simulink model "ddc_bpm_476_066"  (Simulink 7.8)
settings: Solver=ode45  StartTime=0.0  StopTime=2e-3  RelTol=1e-3
undefined symbols (not defined in the file): decim_factor_poly_35, dt_sim, frev_476, Fs_adc, n_ch, n_ovs, R_fofb, R_sec, R_sec_cfir, R_sec_pfir, R_tbt, xlipgetpartsetting
libraries: xbsIndex_r4 x1408, simulink x7
(part 5 of 11)

== system ddc_bpm_476_066/K_monit_mult3/Cast_truncate1 ==
  In1 : Inport
  Reinterpret : xbsIndex_r4/Reinterpret  force_arith_type=on  arith_type="Signed  (2's comp)"  force_bin_pt=on  bin_pt=0  block_type=reinterpret
  Slice : xbsIndex_r4/Slice  nbits=26  boolean_output=off  mode=Upper Bit Location + Width  bit1=0  base1=MSB of Input  bit0=0  base0=LSB of Input  dbl_ovrd=off  block_type=slice
  Out1 : Outport
  wires:
  Slice/1 -> Reinterpret/1
  Reinterpret/1 -> Out1/1
  In1/1 -> Slice/1

== system ddc_bpm_476_066/K_monit_mult4/Cast_truncate1 ==
  In1 : Inport
  Reinterpret : xbsIndex_r4/Reinterpret  force_arith_type=on  arith_type="Signed  (2's comp)"  force_bin_pt=on  bin_pt=0  block_type=reinterpret
  Slice : xbsIndex_r4/Slice  nbits=26  boolean_output=off  mode=Upper Bit Location + Width  bit1=0  base1=MSB of Input  bit0=0  base0=LSB of Input  dbl_ovrd=off  block_type=slice
  Out1 : Outport
  wires:
  Slice/1 -> Reinterpret/1
  Reinterpret/1 -> Out1/1
  In1/1 -> Slice/1

== system ddc_bpm_476_066/K_monit_mult5/Cast_truncate1 ==
  In1 : Inport
  Reinterpret : xbsIndex_r4/Reinterpret  force_arith_type=on  arith_type="Signed  (2's comp)"  force_bin_pt=on  bin_pt=0  block_type=reinterpret
  Slice : xbsIndex_r4/Slice  nbits=26  boolean_output=off  mode=Upper Bit Location + Width  bit1=0  base1=MSB of Input  bit0=0  base0=LSB of Input  dbl_ovrd=off  block_type=slice
  Out1 : Outport
  wires:
  Slice/1 -> Reinterpret/1
  Reinterpret/1 -> Out1/1
  In1/1 -> Slice/1

== system ddc_bpm_476_066/K_tbt_mult/Cast_truncate1 ==
  In1 : Inport
  Reinterpret : xbsIndex_r4/Reinterpret  force_arith_type=on  arith_type="Signed  (2's comp)"  force_bin_pt=on  bin_pt=0  block_type=reinterpret
  Slice : xbsIndex_r4/Slice  nbits=26  boolean_output=off  mode=Upper Bit Location + Width  bit1=0  base1=MSB of Input  bit0=0  base0=LSB of Input  dbl_ovrd=off  block_type=slice
  Out1 : Outport
  wires:
  Slice/1 -> Reinterpret/1
  Reinterpret/1 -> Out1/1
  In1/1 -> Slice/1

== system ddc_bpm_476_066/K_tbt_mult1/Cast_truncate1 ==
  In1 : Inport
  Reinterpret : xbsIndex_r4/Reinterpret  force_arith_type=on  arith_type="Signed  (2's comp)"  force_bin_pt=on  bin_pt=0  block_type=reinterpret
  Slice : xbsIndex_r4/Slice  nbits=26  boolean_output=off  mode=Upper Bit Location + Width  bit1=0  base1=MSB of Input  bit0=0  base0=LSB of Input  dbl_ovrd=off  block_type=slice
  Out1 : Outport
  wires:
  Slice/1 -> Reinterpret/1
  Reinterpret/1 -> Out1/1
  In1/1 -> Slice/1

== system ddc_bpm_476_066/K_tbt_mult2/Cast_truncate1 ==
  In1 : Inport
  Reinterpret : xbsIndex_r4/Reinterpret  force_arith_type=on  arith_type="Signed  (2's comp)"  force_bin_pt=on  bin_pt=0  block_type=reinterpret
  Slice : xbsIndex_r4/Slice  nbits=26  boolean_output=off  mode=Upper Bit Location + Width  bit1=0  base1=MSB of Input  bit0=0  base0=LSB of Input  dbl_ovrd=off  block_type=slice
  Out1 : Outport
  wires:
  Slice/1 -> Reinterpret/1
  Reinterpret/1 -> Out1/1
  In1/1 -> Slice/1

== system ddc_bpm_476_066/Ksum_fofb_mult4/Cast_truncate1 ==
  In1 : Inport
  Reinterpret : xbsIndex_r4/Reinterpret  force_arith_type=on  arith_type="Signed  (2's comp)"  force_bin_pt=on  bin_pt=20  block_type=reinterpret
  Slice : xbsIndex_r4/Slice  nbits=26  boolean_output=off  mode=Upper Bit Location + Width  bit1=0  base1=MSB of Input  bit0=0  base0=LSB of Input  dbl_ovrd=off  block_type=slice
  Out1 : Outport
  wires:
  Slice/1 -> Reinterpret/1
  Reinterpret/1 -> Out1/1
  In1/1 -> Slice/1

== system ddc_bpm_476_066/Ksum_monit_1_mult1/Cast_truncate1 ==
  In1 : Inport
  Reinterpret : xbsIndex_r4/Reinterpret  force_arith_type=on  arith_type="Signed  (2's comp)"  force_bin_pt=on  bin_pt=20  block_type=reinterpret
  Slice : xbsIndex_r4/Slice  nbits=26  boolean_output=off  mode=Upper Bit Location + Width  bit1=0  base1=MSB of Input  bit0=0  base0=LSB of Input  dbl_ovrd=off  block_type=slice
  Out1 : Outport
  wires:
  Slice/1 -> Reinterpret/1
  Reinterpret/1 -> Out1/1
  In1/1 -> Slice/1

== system ddc_bpm_476_066/Ksum_monit_mult2/Cast_truncate1 ==
  In1 : Inport
  Reinterpret : xbsIndex_r4/Reinterpret  force_arith_type=on  arith_type="Signed  (2's comp)"  force_bin_pt=on  bin_pt=20  block_type=reinterpret
  Slice : xbsIndex_r4/Slice  nbits=26  boolean_output=off  mode=Upper Bit Location + Width  bit1=0  base1=MSB of Input  bit0=0  base0=LSB of Input  dbl_ovrd=off  block_type=slice
  Out1 : Outport
  wires:
  Slice/1 -> Reinterpret/1
  Reinterpret/1 -> Out1/1
  In1/1 -> Slice/1

== system ddc_bpm_476_066/Ksum_tbt_mult3/Cast_truncate1 ==
  In1 : Inport
  Reinterpret : xbsIndex_r4/Reinterpret  force_arith_type=on  arith_type="Signed  (2's comp)"  force_bin_pt=on  bin_pt=20  block_type=reinterpret
  Slice : xbsIndex_r4/Slice  nbits=26  boolean_output=off  mode=Upper Bit Location + Width  bit1=0  base1=MSB of Input  bit0=0  base0=LSB of Input  dbl_ovrd=off  block_type=slice
  Out1 : Outport
  wires:
  Slice/1 -> Reinterpret/1
  Reinterpret/1 -> Out1/1
  In1/1 -> Slice/1

== system ddc_bpm_476_066/Mixer/CMixer_0 ==
  din_q : Inport
  din_i : Inport  Port=2
  en : Inport  Port=3
  dds_valid : Inport  Port=4
  dds_msine : Inport  Port=5
  dds_cosine : Inport  Port=6
  ch_in : Inport  Port=7
  ComplexMult : xbsIndex_r4/Complex Multiplier 5.0   hasatlast=off  hasatuser=off  atuserwidth=1  hasbtlast=off  hasbtuser=on  btuserwidth=ceil(log2(n_ovs))  multtype=Use_Mults  optimizegoal=Performance  flowcontrol=NonBlocking  outputwidth=24  roundmode=Truncate  hasctrltlast=off  hasctrltuser=off  ctrltuserwidth=1  outtlastbehv=Null  latencyconfig=Automatic  minimumlatency=34  aclken=off  aresetn=off  trim_axipin_name=on  aportwidth=63  bportwidth=63  ip_name=Complex Multiplier  ip_version=5.0  dsptool_ready=true  ipcore_usecache=true  ipcore_useipmodelcache=true  ipcore_verbose=false  ipcore_latency_parameter='minimumlatency'  wrapper_available=true  port_translation_map={ 'aclken' => 'en', 'aresetn' => 'rst'}  structural_sim=false  block_type=cmpy_v5_0
  Convert1 : xbsIndex_r4/Convert  gui_display_data_type=Fixed-point  arith_type="Signed  (2's comp)"  n_bits=24  bin_pt=22  float_type=Single  exp_bits=8  fraction_bits=24  quantization=Truncate  overflow=Flag as error  en=off  latency=0  dbl_ovrd=off  pipeline=off  block_type=convert
  Convert2 : xbsIndex_r4/Convert  gui_display_data_type=Fixed-point  arith_type="Signed  (2's comp)"  n_bits=24  bin_pt=22  float_type=Single  exp_bits=8  fraction_bits=24  quantization=Truncate  overflow=Flag as error  en=off  latency=0  dbl_ovrd=off  pipeline=off  block_type=convert
  DataReg_En : Subsystem
  DataReg_En1 : Subsystem
  Delay : xbsIndex_r4/Delay  rst=off  infoeditControl=Selection of Reset will increase slice count due to use of real FFs and instead of SRLs  en=off  latency=0  dbl_ovrd=off  reg_retiming=off  block_type=delay
      settings: infoedit=Hardware notes: A delay line is a chain, each link of which is an SRL16 followed by a flip-flop. If register retiming is enabled, the delay line is a chain of flip-flops.  xl_area=[7 14 0 0 0 0 0]  block_version=VER_STRING_GOES_HERE
  Delay1 : xbsIndex_r4/Delay  rst=off  infoeditControl=Selection of Reset will increase slice count due to use of real FFs and instead of SRLs  en=off  latency=0  dbl_ovrd=off  reg_retiming=off  block_type=delay
      settings: infoedit=Hardware notes: A delay line is a chain, each link of which is an SRL16 followed by a flip-flop. If register retiming is enabled, the delay line is a chain of flip-flops.  xl_area=[7 14 0 0 0 0 0]  block_version=VER_STRING_GOES_HERE
  Register{,1..5} (6 alike) : xbsIndex_r4/Register  init=0  rst=off  en=on  dbl_ovrd=off  block_type=register
      settings: block_version=VER_STRING_GOES_HERE
  Register6 : xbsIndex_r4/Register  init=0  rst=off  en=off  dbl_ovrd=off  block_type=register
      settings: block_version=VER_STRING_GOES_HERE
  Reinterpret : xbsIndex_r4/Reinterpret  force_arith_type=off  arith_type=Unsigned  force_bin_pt=off  bin_pt=22  block_type=reinterpret
  Reinterpret1 : xbsIndex_r4/Reinterpret  force_arith_type=off  arith_type=Unsigned  force_bin_pt=off  bin_pt=22  block_type=reinterpret
  Terminator : Terminator
  Q_out : Outport
  I_out : Outport  Port=2
  ch_out : Outport  Port=3
  vout : Outport  Port=4
  wires:
  DataReg_En/1(Dout) -> Delay/1
  DataReg_En1/1(Dout) -> Delay1/1
  dds_cosine/1 -> Register1/1
  dds_msine/1 -> Register2/1
  Register1/1 -> ComplexMult/3  "a_r"
  Register5/1 -> Q_out/1
  Register2/1 -> ComplexMult/2  "a_i"
  ComplexMult/2 -> Reinterpret/1
  ComplexMult/3 -> Reinterpret1/1
  ComplexMult/1 -> Register3/2, Register4/2, Register5/2, Register6/1
  Delay1/1 -> ComplexMult/6  "b_r"
  Delay/1 -> ComplexMult/5  "b_i"
  DataReg_En/2(Valid) -> ComplexMult/4
  Register4/1 -> I_out/1
  Convert1/1 -> Register4/1
  Convert2/1 -> Register5/1
  Reinterpret/1 -> Convert2/1
  Reinterpret1/1 -> Convert1/1
  dds_valid/1 -> Register1/2, Register2/2, ComplexMult/1
  din_q/1 -> DataReg_En/1(Din)
  din_i/1 -> DataReg_En1/1(Din)
  en/1 -> DataReg_En/2(en), DataReg_En1/2(en), Register/2
  ch_in/1 -> Register/1
  Register/1 -> ComplexMult/7
  Register3/1 -> ch_out/1
  ComplexMult/4 -> Register3/1
  Register6/1 -> vout/1
  DataReg_En1/2(Valid) -> Terminator/1

== system ddc_bpm_476_066/Mixer/CMixer_1 ==
  din_q : Inport
  din_i : Inport  Port=2
  en : Inport  Port=3
  dds_valid : Inport  Port=4
  dds_msine : Inport  Port=5
  dds_cosine : Inport  Port=6
  ch_in : Inport  Port=7
  ComplexMult : xbsIndex_r4/Complex Multiplier 5.0   hasatlast=off  hasatuser=off  atuserwidth=1  hasbtlast=off  hasbtuser=on  btuserwidth=ceil(log2(n_ovs))  multtype=Use_Mults  optimizegoal=Performance  flowcontrol=NonBlocking  outputwidth=24  roundmode=Truncate  hasctrltlast=off  hasctrltuser=off  ctrltuserwidth=1  outtlastbehv=Null  latencyconfig=Automatic  minimumlatency=34  aclken=off  aresetn=off  trim_axipin_name=on  aportwidth=63  bportwidth=63  ip_name=Complex Multiplier  ip_version=5.0  dsptool_ready=true  ipcore_usecache=true  ipcore_useipmodelcache=true  ipcore_verbose=false  ipcore_latency_parameter='minimumlatency'  wrapper_available=true  port_translation_map={ 'aclken' => 'en', 'aresetn' => 'rst'}  structural_sim=false  block_type=cmpy_v5_0
  Convert1 : xbsIndex_r4/Convert  gui_display_data_type=Fixed-point  arith_type="Signed  (2's comp)"  n_bits=24  bin_pt=22  float_type=Single  exp_bits=8  fraction_bits=24  quantization=Truncate  overflow=Flag as error  en=off  latency=0  dbl_ovrd=off  pipeline=off  block_type=convert
  Convert2 : xbsIndex_r4/Convert  gui_display_data_type=Fixed-point  arith_type="Signed  (2's comp)"  n_bits=24  bin_pt=22  float_type=Single  exp_bits=8  fraction_bits=24  quantization=Truncate  overflow=Flag as error  en=off  latency=0  dbl_ovrd=off  pipeline=off  block_type=convert
  DataReg_En : Subsystem
  DataReg_En1 : Subsystem
  Delay : xbsIndex_r4/Delay  rst=off  infoeditControl=Selection of Reset will increase slice count due to use of real FFs and instead of SRLs  en=off  latency=0  dbl_ovrd=off  reg_retiming=off  block_type=delay
      settings: infoedit=Hardware notes: A delay line is a chain, each link of which is an SRL16 followed by a flip-flop. If register retiming is enabled, the delay line is a chain of flip-flops.  xl_area=[7 14 0 0 0 0 0]  block_version=VER_STRING_GOES_HERE
  Delay1 : xbsIndex_r4/Delay  rst=off  infoeditControl=Selection of Reset will increase slice count due to use of real FFs and instead of SRLs  en=off  latency=0  dbl_ovrd=off  reg_retiming=off  block_type=delay
      settings: infoedit=Hardware notes: A delay line is a chain, each link of which is an SRL16 followed by a flip-flop. If register retiming is enabled, the delay line is a chain of flip-flops.  xl_area=[7 14 0 0 0 0 0]  block_version=VER_STRING_GOES_HERE
  Register{,1..5} (6 alike) : xbsIndex_r4/Register  init=0  rst=off  en=on  dbl_ovrd=off  block_type=register
      settings: block_version=VER_STRING_GOES_HERE
  Register6 : xbsIndex_r4/Register  init=0  rst=off  en=off  dbl_ovrd=off  block_type=register
      settings: block_version=VER_STRING_GOES_HERE
  Reinterpret : xbsIndex_r4/Reinterpret  force_arith_type=off  arith_type=Unsigned  force_bin_pt=off  bin_pt=22  block_type=reinterpret
  Reinterpret1 : xbsIndex_r4/Reinterpret  force_arith_type=off  arith_type=Unsigned  force_bin_pt=off  bin_pt=22  block_type=reinterpret
  Terminator : Terminator
  Q_out : Outport
  I_out : Outport  Port=2
  ch_out : Outport  Port=3
  vout : Outport  Port=4
  wires:
  DataReg_En/1(Dout) -> Delay/1
  DataReg_En1/1(Dout) -> Delay1/1
  dds_cosine/1 -> Register1/1
  dds_msine/1 -> Register2/1
  Register1/1 -> ComplexMult/3  "a_r"
  Register5/1 -> Q_out/1
  Register2/1 -> ComplexMult/2  "a_i"
  ComplexMult/2 -> Reinterpret/1
  ComplexMult/3 -> Reinterpret1/1
  ComplexMult/1 -> Register3/2, Register4/2, Register5/2, Register6/1
  Delay1/1 -> ComplexMult/6  "b_r"
  Delay/1 -> ComplexMult/5  "b_i"
  DataReg_En/2(Valid) -> ComplexMult/4
  Register4/1 -> I_out/1
  Convert1/1 -> Register4/1
  Convert2/1 -> Register5/1
  Reinterpret/1 -> Convert2/1
  Reinterpret1/1 -> Convert1/1
  dds_valid/1 -> Register1/2, Register2/2, ComplexMult/1
  din_q/1 -> DataReg_En/1(Din)
  din_i/1 -> DataReg_En1/1(Din)
  en/1 -> DataReg_En/2(en), DataReg_En1/2(en), Register/2
  ch_in/1 -> Register/1
  Register/1 -> ComplexMult/7
  Register3/1 -> ch_out/1
  ComplexMult/4 -> Register3/1
  Register6/1 -> vout/1
  DataReg_En1/2(Valid) -> Terminator/1

== system ddc_bpm_476_066/Mixer/ST5 ==
  In : Inport
  Display : Display
  Sample Time : xbsIndex_r4/Sample Time  block_type=sampletime
      settings: infoedit="The Sample Time block reports the normalized sample period of its input.  A signal's normalized sample period is not equivalent to its Simulink absolute sample period.<br><br>Hardware notes: This block is implemented as a constant in hardware."
  out : xbsIndex_r4/Gateway Out  inherit_from_input=on  hdl_port=off  timing_constraint=Data Rate  locs_specified=off  LOCs={}  UseAsDAC=off  DACChannel='1'  block_type=gatewayout
      settings: infoedit="Gateway out block.  Converts Xilinx fixed-point or floating-point type inputs into ouputs of type Simulink integer, single, double, or fixed point.<br><br>Hardware notes:  In hardware these blocks become top level output ports or are discarded, depending on how they are configured."
  wires:
  out/1 -> Display/1
  Sample Time/1 -> out/1
  In/1 -> Sample Time/1

== system ddc_bpm_476_066/Mixer/TDDM_Mixer ==
  mix0_q_in : Inport
  mix0_i_in : Inport  Port=2
  mix0_ch_in : Inport  Port=3
  mix1_q_in : Inport  Port=4
  mix1_i_in : Inport  Port=5
  mix1_ch_in : Inport  Port=6
  TDDM_Mixer0_i : Subsystem
  TDDM_Mixer0_q : Subsystem
  TDDM_Mixer1_i : Subsystem
  TDDM_Mixer1_q : Subsystem
  Terminator{,1..3} (4 alike) : Terminator
  mix_ch0_q_out : Outport
  mix_ch1_q_out : Outport  Port=2
  mix_ch2_q_out : Outport  Port=3
  mix_ch3_q_out : Outport  Port=4
  mix_ch0_i_out : Outport  Port=5
  mix_ch1_i_out : Outport  Port=6
  mix_ch2_i_out : Outport  Port=7
  mix_ch3_i_out : Outport  Port=8
  wires:
  mix0_q_in/1 -> TDDM_Mixer0_q/1(din)
  mix0_ch_in/1 -> TDDM_Mixer0_q/2(ch_in), TDDM_Mixer0_i/2(ch_in)
  mix0_i_in/1 -> TDDM_Mixer0_i/1(din)
  mix1_q_in/1 -> TDDM_Mixer1_q/1(din)
  mix1_ch_in/1 -> TDDM_Mixer1_q/2(ch_in), TDDM_Mixer1_i/2(ch_in)
  mix1_i_in/1 -> TDDM_Mixer1_i/1(din)
  TDDM_Mixer0_q/1(dout_ch0) -> mix_ch0_q_out/1
  TDDM_Mixer0_q/2(dout_ch1) -> mix_ch1_q_out/1
  TDDM_Mixer0_i/1(dout_ch0) -> mix_ch0_i_out/1
  TDDM_Mixer0_i/2(dout_ch1) -> mix_ch1_i_out/1
  TDDM_Mixer1_q/1(dout_ch0) -> mix_ch2_q_out/1
  TDDM_Mixer1_q/2(dout_ch1) -> mix_ch3_q_out/1
  TDDM_Mixer1_i/1(dout_ch0) -> mix_ch2_i_out/1
  TDDM_Mixer1_i/2(dout_ch1) -> mix_ch3_i_out/1
  TDDM_Mixer0_i/3(ch_out) -> Terminator/1
  TDDM_Mixer0_q/3(ch_out) -> Terminator1/1
  TDDM_Mixer1_i/3(ch_out) -> Terminator2/1
  TDDM_Mixer1_q/3(ch_out) -> Terminator3/1

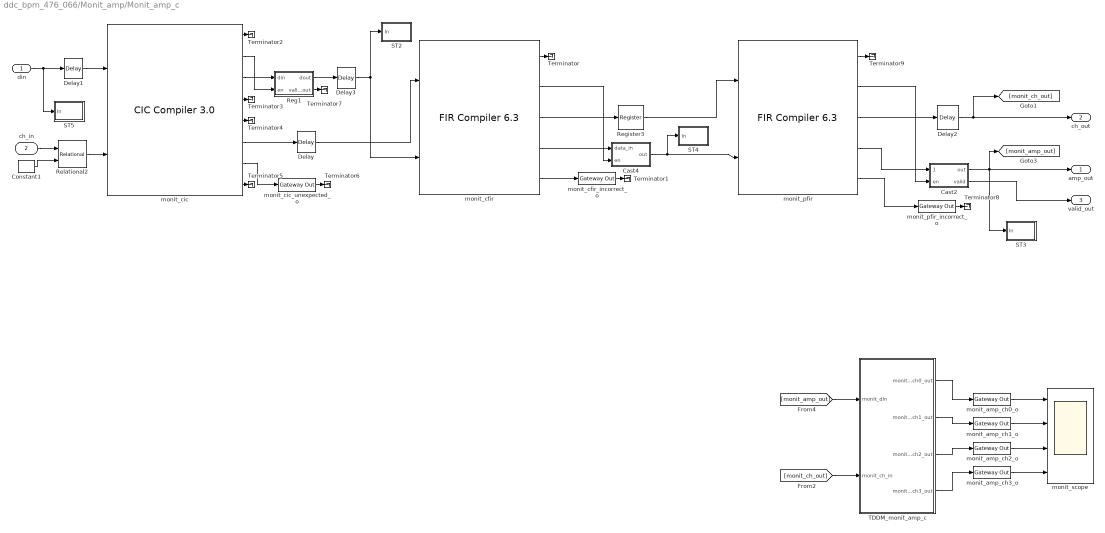
== system ddc_bpm_476_066/Monit_amp/Monit_amp_c ==
  din : Inport
  ch_in : Inport  Port=2
  Cast2 : Subsystem
  Cast4 : Subsystem
  Constant1 : xbsIndex_r4/Constant  const=2  gui_display_data_type=Fixed-point  arith_type=Unsigned  n_bits=2  bin_pt=0  preci_type=Single  exp_width=8  frac_width=24  explicit_period=off  period=1  equ=P=C  opselect=C  inp2=PCIN>>17  opr=+  inp1=P  carry=CIN  dbl_ovrd=off  block_type=constant
  Delay : xbsIndex_r4/Delay  rst=off  infoeditControl=Selection of Reset will increase slice count due to use of real FFs and instead of SRLs  en=off  latency=3  dbl_ovrd=off  reg_retiming=off  block_type=delay
  Delay1 : xbsIndex_r4/Delay  rst=off  infoeditControl=Selection of Reset will increase slice count due to use of real FFs and instead of SRLs  en=off  latency=3  dbl_ovrd=off  reg_retiming=off  block_type=delay
  Delay2 : xbsIndex_r4/Delay  rst=off  infoeditControl=Selection of Reset will increase slice count due to use of real FFs and instead of SRLs  en=off  latency=1  dbl_ovrd=off  reg_retiming=off  block_type=delay
  Delay3 : xbsIndex_r4/Delay  rst=off  infoeditControl=Selection of Reset will increase slice count due to use of real FFs and instead of SRLs  en=off  latency=2  dbl_ovrd=off  reg_retiming=off  block_type=delay
  Reg1 : Subsystem
  Register3 : xbsIndex_r4/Register  init=0  rst=off  en=off  dbl_ovrd=off  block_type=register
      settings: xl_area=[0, 0, 0, 0, 0, 0, 0]  block_version=VER_STRING_GOES_HERE
  Relational2 : xbsIndex_r4/Relational  mode=a=b  en=off  latency=4  dbl_ovrd=off  block_type=relational
  ST2 : Subsystem
  ST3 : Subsystem
  ST4 : Subsystem
  ST5 : Subsystem
  TDDM_monit_amp_c : Subsystem
  Terminator{,1..9} (10 alike) : Terminator
  monit_amp_ch0_o : xbsIndex_r4/Gateway Out  inherit_from_input=on  hdl_port=on  timing_constraint=Data Rate  locs_specified=off  LOCs={}  UseAsDAC=off  DACChannel='1'  block_type=gatewayout
      settings: infoedit="Gateway out block.  Converts Xilinx fixed-point or floating-point type inputs into ouputs of type Simulink integer, single, double, or fixed point.<br><br>Hardware notes:  In hardware these blocks become top level output ports or are discarded, depending on how they are configured."
  monit_amp_ch1_o : xbsIndex_r4/Gateway Out  inherit_from_input=on  hdl_port=on  timing_constraint=Data Rate  locs_specified=off  LOCs={}  UseAsDAC=off  DACChannel='1'  block_type=gatewayout
      settings: infoedit="Gateway out block.  Converts Xilinx fixed-point or floating-point type inputs into ouputs of type Simulink integer, single, double, or fixed point.<br><br>Hardware notes:  In hardware these blocks become top level output ports or are discarded, depending on how they are configured."
  monit_amp_ch2_o : xbsIndex_r4/Gateway Out  inherit_from_input=on  hdl_port=on  timing_constraint=Data Rate  locs_specified=off  LOCs={}  UseAsDAC=off  DACChannel='1'  block_type=gatewayout
      settings: infoedit="Gateway out block.  Converts Xilinx fixed-point or floating-point type inputs into ouputs of type Simulink integer, single, double, or fixed point.<br><br>Hardware notes:  In hardware these blocks become top level output ports or are discarded, depending on how they are configured."
  monit_amp_ch3_o : xbsIndex_r4/Gateway Out  inherit_from_input=on  hdl_port=on  timing_constraint=Data Rate  locs_specified=off  LOCs={}  UseAsDAC=off  DACChannel='1'  block_type=gatewayout
      settings: infoedit="Gateway out block.  Converts Xilinx fixed-point or floating-point type inputs into ouputs of type Simulink integer, single, double, or fixed point.<br><br>Hardware notes:  In hardware these blocks become top level output ports or are discarded, depending on how they are configured."
  monit_cfir : xbsIndex_r4/FIR Compiler 6.3   coefficientvector=hcfir_sec.Numerator  coefficient_sets=1  coefficient_reload=off  filter_type=Decimation  rate_change_type=Integer  interpolation_rate=1  decimation_rate=R_sec_cfir  zero_pack_factor=1  channel_sequence=Basic  number_channels=4  pattern_list='P4-0,P4-1,P4-2,P4-3,P4-4'  number_paths=1  ratespecification=Hardware_Oversampling_Rate  sampleperiod=1  hardwareoversamplingrate=R_fofb*R_sec*n_ovs/n_ch  coefficient_sign=Signed  quantization=Quantize_Only  coefficient_width=16  bestprecision=on  coefficient_fractional_bits=15  coefficient_structure=Inferred  output_rounding_mode=Convergent_Rounding_to_Even  output_width=25  filter_architecture=Systolic_Multiply_Accumulate  optimization_goal=Area  data_buffer_type=Automatic  coefficient_buffer_type=Automatic  input_buffer_type=Automatic  output_buffer_type=Automatic  preference_for_other_storage=Automatic  multi_column_support=Automatic  columnconfig='1'  inter_column_pipe_length=4  data_has_tlast=Not_Required  m_data_has_tready=off  s_data_has_fifo=off  s_data_has_tuser=Chan_ID_Field  m_data_has_tuser=Chan_ID_Field  s_config_sync_mode=On_Vector  s_config_method=Single  num_reload_slots=1  has_aclken=off  has_aresetn=off  infoeditControl=ARESETn must be asserted for a minmum of 2 cycles  trim_axipin_name=on  passband_min=0.0  passband_max=0.5  stopband_min=0.5  stopband_max=1.0  filter_selection=1  gui_behaviour=Sysgen_GUI  data_sign=Signed  data_width=16  data_fractional_bits=0  data_tuser_width=1  wrapper_available=true  ip_wrap_arbitrary_binary_point=true  simulation_type=external_xfix  simulation_model=firv6_3_CModel:firv6_3_cmodel  ip_name=FIR Compiler  ip_version=6.3  dsptool_ready=true  ipcore_usecache=true  ipcore_useipmodelcache=true  ipcore_xco_need_fpga_part=true  port_translation_map={ 'aclken' => 'en', 'aresetn' => 'rst' }  run_core_at_system_period=true  ipcore_fpga_part=xlipgetpartsetting(gcb, {'virtex6', 'xc6vlx75t', '-3', 'ff784'})  block_type=fir_compiler_v6_3
      settings: infoedit=Maximum Possible : Maximizes oversampling rate. Abstracted input handshake (no s_data_tvalid) and automatic rate propagation.<br>Hardware Oversampling Rate : Specifies oversampling rate relative to the input sample period. Abstracted input handshake (no s_data_tvalid) and automatic rate propagation.<br>Sample Period : Specifies absolute oversampling rate. No input handshake abstraction (exposes s_data_tvalid) and no rate propagation.
  monit_cfir_incorrect_o : xbsIndex_r4/Gateway Out  inherit_from_input=on  hdl_port=on  timing_constraint=Data Rate  locs_specified=off  LOCs={}  UseAsDAC=off  DACChannel='1'  block_type=gatewayout
      settings: infoedit="Gateway out block.  Converts Xilinx fixed-point or floating-point type inputs into ouputs of type Simulink integer, single, double, or fixed point.<br><br>Hardware notes:  In hardware these blocks become top level output ports or are discarded, depending on how they are configured."
  monit_cic : xbsIndex_r4/CIC Compiler 3.0   filter_type=Decimation  number_of_stages=3  differential_delay=2  number_of_channels=4  sample_rate_changes=Fixed  fixed_or_initial_rate=R_sec  minimum_rate=2500  maximum_rate=2500  ratespecification=Hardware_Oversampling_Rate  sampleperiod=1  hardwareoversamplingrate=R_fofb*n_ovs/n_ch  quantization=Full_Precision  output_data_width=55  use_xtreme_dsp_slice=on  use_streaming_interface=on  has_aclken=off  has_aresetn=off  has_dout_tready=off  trim_axipin_name=on  gui_behaviour=Sysgen_GUI  input_data_width=18  ip_name=CIC Compiler  ip_version=3.0  dsptool_ready=true  wrapper_available=true  port_translation_map={ 'aclken' => 'en', 'aresetn' => 'rst' }  ipcore_xco_need_fpga_part=true  ipcore_fpga_part=xlipgetpartsetting(gcb, {'virtex7', 'xc7v1500t', '-2', 'fhg1157'})  ipcore_verbose=false  block_type=cic_compiler_v3_0
  monit_cic_unexpected_o : xbsIndex_r4/Gateway Out  inherit_from_input=on  hdl_port=on  timing_constraint=Data Rate  locs_specified=off  LOCs={}  UseAsDAC=off  DACChannel='1'  block_type=gatewayout
      settings: infoedit="Gateway out block.  Converts Xilinx fixed-point or floating-point type inputs into ouputs of type Simulink integer, single, double, or fixed point.<br><br>Hardware notes:  In hardware these blocks become top level output ports or are discarded, depending on how they are configured."
  monit_pfir : xbsIndex_r4/FIR Compiler 6.3   coefficientvector=hpfir_sec.Numerator  coefficient_sets=1  coefficient_reload=off  filter_type=Decimation  rate_change_type=Integer  interpolation_rate=1  decimation_rate=R_sec_pfir  zero_pack_factor=1  channel_sequence=Basic  number_channels=4  pattern_list='P4-0,P4-1,P4-2,P4-3,P4-4'  number_paths=1  ratespecification=Hardware_Oversampling_Rate  sampleperiod=1  hardwareoversamplingrate=R_fofb*R_sec*R_sec_cfir*n_ovs/n_ch  coefficient_sign=Signed  quantization=Quantize_Only  coefficient_width=16  bestprecision=on  coefficient_fractional_bits=15  coefficient_structure=Inferred  output_rounding_mode=Convergent_Rounding_to_Even  output_width=25  filter_architecture=Systolic_Multiply_Accumulate  optimization_goal=Area  data_buffer_type=Automatic  coefficient_buffer_type=Automatic  input_buffer_type=Automatic  output_buffer_type=Automatic  preference_for_other_storage=Automatic  multi_column_support=Automatic  columnconfig='1'  inter_column_pipe_length=4  data_has_tlast=Not_Required  m_data_has_tready=off  s_data_has_fifo=off  s_data_has_tuser=Chan_ID_Field  m_data_has_tuser=Chan_ID_Field  s_config_sync_mode=On_Vector  s_config_method=Single  num_reload_slots=1  has_aclken=off  has_aresetn=off  infoeditControl=ARESETn must be asserted for a minmum of 2 cycles  trim_axipin_name=on  passband_min=0.0  passband_max=0.5  stopband_min=0.5  stopband_max=1.0  filter_selection=1  gui_behaviour=Sysgen_GUI  data_sign=Signed  data_width=16  data_fractional_bits=0  data_tuser_width=1  wrapper_available=true  ip_wrap_arbitrary_binary_point=true  simulation_type=external_xfix  simulation_model=firv6_3_CModel:firv6_3_cmodel  ip_name=FIR Compiler  ip_version=6.3  dsptool_ready=true  ipcore_usecache=true  ipcore_useipmodelcache=true  ipcore_xco_need_fpga_part=true  port_translation_map={ 'aclken' => 'en', 'aresetn' => 'rst' }  run_core_at_system_period=true  ipcore_fpga_part=xlipgetpartsetting(gcb, {'virtex6', 'xc6vlx75t', '-3', 'ff784'})  block_type=fir_compiler_v6_3
      settings: infoedit=Maximum Possible : Maximizes oversampling rate. Abstracted input handshake (no s_data_tvalid) and automatic rate propagation.<br>Hardware Oversampling Rate : Specifies oversampling rate relative to the input sample period. Abstracted input handshake (no s_data_tvalid) and automatic rate propagation.<br>Sample Period : Specifies absolute oversampling rate. No input handshake abstraction (exposes s_data_tvalid) and no rate propagation.
  monit_pfir_incorrect_o : xbsIndex_r4/Gateway Out  inherit_from_input=on  hdl_port=on  timing_constraint=Data Rate  locs_specified=off  LOCs={}  UseAsDAC=off  DACChannel='1'  block_type=gatewayout
      settings: infoedit="Gateway out block.  Converts Xilinx fixed-point or floating-point type inputs into ouputs of type Simulink integer, single, double, or fixed point.<br><br>Hardware notes:  In hardware these blocks become top level output ports or are discarded, depending on how they are configured."
  monit_scope : Scope  NumInputPorts=4
      settings: TimeRange=0.00011214  YMin=-0.1~-1.5~-0.002~-1.5  YMax=1~1.5~0.00075~1.5  SaveName=ScopeData2  MaxDataPoints=1000000  SampleInput=on
  amp_out : Outport
  ch_out : Outport  Port=2
  valid_out : Outport  Port=3
  wires:
  din/1 -> ST5/1(In), Delay1/1
  ch_in/1 -> Relational2/1
  Relational2/1 -> monit_cic/2
  monit_cic/3 -> Reg1/1(din)
  monit_cic/2 -> Reg1/2(en)
  monit_cic/6 -> Delay/1
  monit_cic/1 -> Terminator2/1
  monit_cic/4 -> Terminator3/1
  monit_cic/5 -> Terminator4/1
  Reg1/1(dout) -> Delay3/1
  [monit_amp_out] -> TDDM_monit_amp_c/1(monit_din)
  [monit_ch_out] -> TDDM_monit_amp_c/2(monit_ch_in)
  TDDM_monit_amp_c/1(monit_ch0_out) -> monit_amp_ch0_o/1
  TDDM_monit_amp_c/2(monit_ch1_out) -> monit_amp_ch1_o/1
  TDDM_monit_amp_c/3(monit_ch2_out) -> monit_amp_ch2_o/1
  TDDM_monit_amp_c/4(monit_ch3_out) -> monit_amp_ch3_o/1
  monit_amp_ch3_o/1 -> monit_scope/4
  monit_amp_ch2_o/1 -> monit_scope/3
  monit_amp_ch1_o/1 -> monit_scope/2
  monit_amp_ch0_o/1 -> monit_scope/1
  Delay2/1 -> ch_out/1, [monit_ch_out]
  Cast2/1(out) -> amp_out/1, ST3/1(In), [monit_amp_out]
  Cast2/2(valid) -> valid_out/1
  Delay/1 -> monit_cfir/1
  Reg1/2(valid_out) -> Terminator7/1
  monit_cic/7 -> monit_cic_unexpected_o/1
  monit_cic/8 -> Terminator5/1
  Cast4/1(out) -> ST4/1(In), monit_pfir/2
  monit_cfir/3 -> Register3/1
  monit_cfir/4 -> Cast4/1(data_in)
  monit_cfir/2 -> Cast4/2(en)
  Register3/1 -> monit_pfir/1
  monit_pfir/4 -> Cast2/1(data_in)
  monit_pfir/3 -> Delay2/1
  monit_pfir/1 -> Terminator9/1
  monit_pfir/2 -> Cast2/2(en)
  monit_pfir/5 -> monit_pfir_incorrect_o/1
  monit_cfir/5 -> monit_cfir_incorrect_o/1
  monit_cfir/1 -> Terminator/1
  monit_cfir_incorrect_o/1 -> Terminator1/1
  monit_cic_unexpected_o/1 -> Terminator6/1
  monit_pfir_incorrect_o/1 -> Terminator8/1
  Constant1/1 -> Relational2/2
  Delay1/1 -> monit_cic/1
  Delay3/1 -> ST2/1(In), monit_cfir/2

== system ddc_bpm_476_066/Monit_amp/TDDM_monit_amp_out ==
  monit_amp_din : Inport
  monit_amp_ch_in : Inport  Port=2
  TDDM_monit_amp_out_int : Subsystem
  Terminator : Terminator
  monit_amp_data0_out : Outport
  monit_amp_data1_out : Outport  Port=2
  monit_amp_data2_out : Outport  Port=3
  monit_amp_data3_out : Outport  Port=4
  wires:
  TDDM_monit_amp_out_int/1(dout_ch0) -> monit_amp_data0_out/1
  TDDM_monit_amp_out_int/2(dout_ch1) -> monit_amp_data1_out/1
  TDDM_monit_amp_out_int/3(dout_ch2) -> monit_amp_data2_out/1
  TDDM_monit_amp_out_int/4(dout_ch3) -> monit_amp_data3_out/1
  monit_amp_din/1 -> TDDM_monit_amp_out_int/1(din)
  monit_amp_ch_in/1 -> TDDM_monit_amp_out_int/2(ch_in)
  TDDM_monit_amp_out_int/5(ch_out) -> Terminator/1

== system ddc_bpm_476_066/TBT_amp/ST5 ==
  In : Inport
  Display : Display
  Sample Time : xbsIndex_r4/Sample Time  block_type=sampletime
      settings: infoedit="The Sample Time block reports the normalized sample period of its input.  A signal's normalized sample period is not equivalent to its Simulink absolute sample period.<br><br>Hardware notes: This block is implemented as a constant in hardware."
  out : xbsIndex_r4/Gateway Out  inherit_from_input=on  hdl_port=off  timing_constraint=Data Rate  locs_specified=off  LOCs={}  UseAsDAC=off  DACChannel='1'  block_type=gatewayout
      settings: infoedit="Gateway out block.  Converts Xilinx fixed-point or floating-point type inputs into ouputs of type Simulink integer, single, double, or fixed point.<br><br>Hardware notes:  In hardware these blocks become top level output ports or are discarded, depending on how they are configured."
  wires:
  out/1 -> Display/1
  Sample Time/1 -> out/1
  In/1 -> Sample Time/1

== system ddc_bpm_476_066/TBT_amp/TBT_amp0 ==
  Q_in : Inport
  I_in : Inport  Port=2
  ch_in : Inport  Port=3
  TBT_CORDIC : Subsystem
  TBT_poly_decim : Subsystem
  amp_out : Outport
  phase_out : Outport  Port=2
  valid_out : Outport  Port=3
  ch_out : Outport  Port=4
  wires:
  Q_in/1 -> TBT_poly_decim/1(Q_in)
  I_in/1 -> TBT_poly_decim/2(I_in)
  ch_in/1 -> TBT_poly_decim/3(ch_in)
  TBT_poly_decim/4(ch_out) -> TBT_CORDIC/4(ch_in)
  TBT_CORDIC/1(amp_out) -> amp_out/1
  TBT_CORDIC/2(phase_out) -> phase_out/1
  TBT_CORDIC/3(valid_out) -> valid_out/1
  TBT_poly_decim/3(valid_out) -> TBT_CORDIC/3(valid_in)
  TBT_poly_decim/2(I_out) -> TBT_CORDIC/2(I_in)
  TBT_poly_decim/1(Q_out) -> TBT_CORDIC/1(Q_in)
  TBT_CORDIC/4(ch_out) -> ch_out/1

== system ddc_bpm_476_066/TBT_amp/TBT_amp1 ==
  Q_in : Inport
  I_in : Inport  Port=2
  ch_in : Inport  Port=3
  TBT_CORDIC : Subsystem
  TBT_poly_decim : Subsystem
  amp_out : Outport
  phase_out : Outport  Port=2
  valid_out : Outport  Port=3
  ch_out : Outport  Port=4
  wires:
  Q_in/1 -> TBT_poly_decim/1(Q_in)
  I_in/1 -> TBT_poly_decim/2(I_in)
  ch_in/1 -> TBT_poly_decim/3(ch_in)
  TBT_CORDIC/1(amp_out) -> amp_out/1
  TBT_CORDIC/2(phase_out) -> phase_out/1
  TBT_CORDIC/3(valid_out) -> valid_out/1
  TBT_CORDIC/4(ch_out) -> ch_out/1
  TBT_poly_decim/1(Q_out) -> TBT_CORDIC/1(Q_in)
  TBT_poly_decim/2(I_out) -> TBT_CORDIC/2(I_in)
  TBT_poly_decim/3(valid_out) -> TBT_CORDIC/3(valid_in)
  TBT_poly_decim/4(ch_out) -> TBT_CORDIC/4(ch_in)

== system ddc_bpm_476_066/TBT_amp/TDDM_tbt_amp_4ch ==
  amp_in0 : Inport
  ch_in0 : Inport  Port=2
  amp_in1 : Inport  Port=3
  ch_in1 : Inport  Port=4
  TDDM_tbt_amp0 : Subsystem
  TDDM_tbt_amp1 : Subsystem
  Terminator : Terminator
  Terminator1 : Terminator
  amp_out0 : Outport
  amp_out1 : Outport  Port=2
  amp_out2 : Outport  Port=3
  amp_out3 : Outport  Port=4
  wires:
  amp_in0/1 -> TDDM_tbt_amp0/1(din)
  ch_in0/1 -> TDDM_tbt_amp0/2(ch_in)
  amp_in1/1 -> TDDM_tbt_amp1/1(din)
  TDDM_tbt_amp0/1(dout_ch0) -> amp_out0/1
  TDDM_tbt_amp0/2(dout_ch1) -> amp_out1/1
  TDDM_tbt_amp1/1(dout_ch0) -> amp_out2/1
  TDDM_tbt_amp1/2(dout_ch1) -> amp_out3/1
  TDDM_tbt_amp1/3(ch_out) -> Terminator/1
  TDDM_tbt_amp0/3(ch_out) -> Terminator1/1
  ch_in1/1 -> TDDM_tbt_amp1/2(ch_in)

== system ddc_bpm_476_066/TDM_mix/ST1 ==
  In : Inport
  Display : Display
  Sample Time : xbsIndex_r4/Sample Time  block_type=sampletime
      settings: infoedit="The Sample Time block reports the normalized sample period of its input.  A signal's normalized sample period is not equivalent to its Simulink absolute sample period.<br><br>Hardware notes: This block is implemented as a constant in hardware."
  out : xbsIndex_r4/Gateway Out  inherit_from_input=on  hdl_port=off  timing_constraint=Data Rate  locs_specified=off  LOCs={}  UseAsDAC=off  DACChannel='1'  block_type=gatewayout
      settings: infoedit="Gateway out block.  Converts Xilinx fixed-point or floating-point type inputs into ouputs of type Simulink integer, single, double, or fixed point.<br><br>Hardware notes:  In hardware these blocks become top level output ports or are discarded, depending on how they are configured."
  wires:
  out/1 -> Display/1
  Sample Time/1 -> out/1
  In/1 -> Sample Time/1

== system ddc_bpm_476_066/TDM_mix/ST2 ==
  In : Inport
  Display : Display
  Sample Time : xbsIndex_r4/Sample Time  block_type=sampletime
      settings: infoedit="The Sample Time block reports the normalized sample period of its input.  A signal's normalized sample period is not equivalent to its Simulink absolute sample period.<br><br>Hardware notes: This block is implemented as a constant in hardware."
  out : xbsIndex_r4/Gateway Out  inherit_from_input=on  hdl_port=off  timing_constraint=Data Rate  locs_specified=off  LOCs={}  UseAsDAC=off  DACChannel='1'  block_type=gatewayout
      settings: infoedit="Gateway out block.  Converts Xilinx fixed-point or floating-point type inputs into ouputs of type Simulink integer, single, double, or fixed point.<br><br>Hardware notes:  In hardware these blocks become top level output ports or are discarded, depending on how they are configured."
  wires:
  out/1 -> Display/1
  Sample Time/1 -> out/1
  In/1 -> Sample Time/1

== system ddc_bpm_476_066/TDM_mix/ST3 ==
  In : Inport
  Display : Display
  Sample Time : xbsIndex_r4/Sample Time  block_type=sampletime
      settings: infoedit="The Sample Time block reports the normalized sample period of its input.  A signal's normalized sample period is not equivalent to its Simulink absolute sample period.<br><br>Hardware notes: This block is implemented as a constant in hardware."
  out : xbsIndex_r4/Gateway Out  inherit_from_input=on  hdl_port=off  timing_constraint=Data Rate  locs_specified=off  LOCs={}  UseAsDAC=off  DACChannel='1'  block_type=gatewayout
      settings: infoedit="Gateway out block.  Converts Xilinx fixed-point or floating-point type inputs into ouputs of type Simulink integer, single, double, or fixed point.<br><br>Hardware notes:  In hardware these blocks become top level output ports or are discarded, depending on how they are configured."
  wires:
  out/1 -> Display/1
  Sample Time/1 -> out/1
  In/1 -> Sample Time/1

== system ddc_bpm_476_066/TDM_mix/ST4 ==
  In : Inport
  Display : Display
  Sample Time : xbsIndex_r4/Sample Time  block_type=sampletime
      settings: infoedit="The Sample Time block reports the normalized sample period of its input.  A signal's normalized sample period is not equivalent to its Simulink absolute sample period.<br><br>Hardware notes: This block is implemented as a constant in hardware."
  out : xbsIndex_r4/Gateway Out  inherit_from_input=on  hdl_port=off  timing_constraint=Data Rate  locs_specified=off  LOCs={}  UseAsDAC=off  DACChannel='1'  block_type=gatewayout
      settings: infoedit="Gateway out block.  Converts Xilinx fixed-point or floating-point type inputs into ouputs of type Simulink integer, single, double, or fixed point.<br><br>Hardware notes:  In hardware these blocks become top level output ports or are discarded, depending on how they are configured."
  wires:
  out/1 -> Display/1
  Sample Time/1 -> out/1
  In/1 -> Sample Time/1

== system ddc_bpm_476_066/TDM_mix/ST5 ==
  In : Inport
  Display : Display
  Sample Time : xbsIndex_r4/Sample Time  block_type=sampletime
      settings: infoedit="The Sample Time block reports the normalized sample period of its input.  A signal's normalized sample period is not equivalent to its Simulink absolute sample period.<br><br>Hardware notes: This block is implemented as a constant in hardware."
  out : xbsIndex_r4/Gateway Out  inherit_from_input=on  hdl_port=off  timing_constraint=Data Rate  locs_specified=off  LOCs={}  UseAsDAC=off  DACChannel='1'  block_type=gatewayout
      settings: infoedit="Gateway out block.  Converts Xilinx fixed-point or floating-point type inputs into ouputs of type Simulink integer, single, double, or fixed point.<br><br>Hardware notes:  In hardware these blocks become top level output ports or are discarded, depending on how they are configured."
  wires:
  out/1 -> Display/1
  Sample Time/1 -> out/1
  In/1 -> Sample Time/1

== system ddc_bpm_476_066/TDM_mix/ST6 ==
  In : Inport
  Display : Display
  Sample Time : xbsIndex_r4/Sample Time  block_type=sampletime
      settings: infoedit="The Sample Time block reports the normalized sample period of its input.  A signal's normalized sample period is not equivalent to its Simulink absolute sample period.<br><br>Hardware notes: This block is implemented as a constant in hardware."
  out : xbsIndex_r4/Gateway Out  inherit_from_input=on  hdl_port=off  timing_constraint=Data Rate  locs_specified=off  LOCs={}  UseAsDAC=off  DACChannel='1'  block_type=gatewayout
      settings: infoedit="Gateway out block.  Converts Xilinx fixed-point or floating-point type inputs into ouputs of type Simulink integer, single, double, or fixed point.<br><br>Hardware notes:  In hardware these blocks become top level output ports or are discarded, depending on how they are configured."
  wires:
  out/1 -> Display/1
  Sample Time/1 -> out/1
  In/1 -> Sample Time/1

== system ddc_bpm_476_066/TDM_mix/TDM_mix_ch0_1 ==
  note: No need for decimation here, as we are at output rate already!
  rst : Inport
  din_ch0 : Inport  Port=2
  din_ch1 : Inport  Port=3
  Clock Enable Probe : xbsIndex_r4/Clock Enable Probe  inherit_constraints=on  block_type=ceprobe
      settings: infoedit="Clock enable extractor.  Produces a Boolean output that mirrors the hardware clock enable associated with the input sample rate.<br><br>Hardware notes: in hardware this block costs nothing."
  D_S3 : Scope  NumInputPorts=4
      settings: TimeRange=0.0004  YMin=-1~-1.5~10~-1.5  YMax=1~1.5~100~1.5  MaxDataPoints=1000000  SampleInput=on
  Gateway Out{,1..2,5} (4 alike) : xbsIndex_r4/Gateway Out  inherit_from_input=on  hdl_port=off  timing_constraint=None  locs_specified=off  LOCs={}  UseAsDAC=off  DACChannel='1'  block_type=gatewayout
      settings: infoedit="Gateway out block.  Converts Xilinx fixed-point or floating-point type inputs into ouputs of type Simulink integer, single, double, or fixed point.<br><br>Hardware notes:  In hardware these blocks become top level output ports or are discarded, depending on how they are configured."
  Mux : xbsIndex_r4/Mux  inputs=2  en=off  latency=0  precision=Full  arith_type=Unsigned  n_bits=16  bin_pt=14  quantization=Truncate  overflow=Wrap  dbl_ovrd=off  block_type=mux
  Register : xbsIndex_r4/Register  init=0  rst=off  en=off  dbl_ovrd=off  block_type=register
  Register1 : xbsIndex_r4/Register  init=0  rst=off  en=off  dbl_ovrd=off  block_type=register
  ST1 : Subsystem
  ST2 : Subsystem
  ST3 : Subsystem
  ST5 : Subsystem
  mux_sel1 : xbsIndex_r4/Counter  cnt_type=Free Running  cnt_to=Inf  operation=Up  start_count=0  cnt_by_val=1  arith_type=Unsigned  n_bits=1  bin_pt=0  load_pin=off  rst=on  en=on  explicit_period=off  period=1/Fs_adc/4*1112  dbl_ovrd=off  use_behavioral_HDL=off  implementation=Fabric  block_type=counter
  up_sample_ch0 : xbsIndex_r4/Up Sample  sample_ratio=n_ch/n_ovs  copy_samples=on  en=off  latency=0  dbl_ovrd=off  block_type=usamp
  up_sample_ch1 : xbsIndex_r4/Up Sample  sample_ratio=n_ch/n_ovs  copy_samples=on  en=off  latency=0  dbl_ovrd=off  block_type=usamp
  dout : Outport
  ch_out : Outport  Port=2
  wires:
  Mux/1 -> Register/1
  up_sample_ch1/1 -> Mux/3, [din_ch1]
  up_sample_ch0/1 -> Mux/2, [din_ch0_up], Clock Enable Probe/1, ST5/1(In)
  rst/1 -> mux_sel1/1
  din_ch0/1 -> up_sample_ch0/1, [din_ch0]
  din_ch1/1 -> up_sample_ch1/1
  Register/1 -> dout/1, [mux_out]
  Register1/1 -> ch_out/1
  [mux_sel] -> Gateway Out/1, ST2/1(In)
  [din_ch0_up] -> Gateway Out1/1, ST1/1(In)
  [din_ch1] -> Gateway Out2/1, ST3/1(In)
  [mux_out] -> Gateway Out5/1
  Gateway Out/1 -> D_S3/1
  Gateway Out1/1 -> D_S3/2
  Gateway Out2/1 -> D_S3/3
  Gateway Out5/1 -> D_S3/4
  mux_sel1/1 -> Register1/1, Mux/1, [mux_sel]
  Clock Enable Probe/1 -> mux_sel1/2

== system ddc_bpm_476_066/TDM_mix/TDM_mix_ch0_2 ==
  note: No need for decimation here, as we are at output rate already!
  rst : Inport
  din_ch0 : Inport  Port=2
  din_ch1 : Inport  Port=3
  Clock Enable Probe : xbsIndex_r4/Clock Enable Probe  inherit_constraints=on  block_type=ceprobe
      settings: infoedit="Clock enable extractor.  Produces a Boolean output that mirrors the hardware clock enable associated with the input sample rate.<br><br>Hardware notes: in hardware this block costs nothing."
  D_S3 : Scope  NumInputPorts=4
      settings: TimeRange=0.0004  YMin=-1~-1.5~10~-1.5  YMax=1~1.5~100~1.5  MaxDataPoints=1000000  SampleInput=on
  Gateway Out{,1..2,5} (4 alike) : xbsIndex_r4/Gateway Out  inherit_from_input=on  hdl_port=off  timing_constraint=None  locs_specified=off  LOCs={}  UseAsDAC=off  DACChannel='1'  block_type=gatewayout
      settings: infoedit="Gateway out block.  Converts Xilinx fixed-point or floating-point type inputs into ouputs of type Simulink integer, single, double, or fixed point.<br><br>Hardware notes:  In hardware these blocks become top level output ports or are discarded, depending on how they are configured."
  Mux : xbsIndex_r4/Mux  inputs=2  en=off  latency=0  precision=Full  arith_type=Unsigned  n_bits=16  bin_pt=14  quantization=Truncate  overflow=Wrap  dbl_ovrd=off  block_type=mux
  Register : xbsIndex_r4/Register  init=0  rst=off  en=off  dbl_ovrd=off  block_type=register
  Register1 : xbsIndex_r4/Register  init=0  rst=off  en=off  dbl_ovrd=off  block_type=register
  ST1 : Subsystem
  ST2 : Subsystem
  ST3 : Subsystem
  ST5 : Subsystem
  mux_sel1 : xbsIndex_r4/Counter  cnt_type=Free Running  cnt_to=Inf  operation=Up  start_count=0  cnt_by_val=1  arith_type=Unsigned  n_bits=1  bin_pt=0  load_pin=off  rst=on  en=on  explicit_period=off  period=1/Fs_adc/4*1112  dbl_ovrd=off  use_behavioral_HDL=off  implementation=Fabric  block_type=counter
  up_sample_ch0 : xbsIndex_r4/Up Sample  sample_ratio=n_ch/n_ovs  copy_samples=on  en=off  latency=0  dbl_ovrd=off  block_type=usamp
  up_sample_ch1 : xbsIndex_r4/Up Sample  sample_ratio=n_ch/n_ovs  copy_samples=on  en=off  latency=0  dbl_ovrd=off  block_type=usamp
  dout : Outport
  ch_out : Outport  Port=2
  wires:
  Mux/1 -> Register/1
  up_sample_ch1/1 -> Mux/3, [din_ch1]
  up_sample_ch0/1 -> Mux/2, [din_ch0_up], Clock Enable Probe/1, ST5/1(In)
  rst/1 -> mux_sel1/1
  din_ch0/1 -> up_sample_ch0/1, [din_ch0]
  din_ch1/1 -> up_sample_ch1/1
  Register/1 -> dout/1, [mux_out]
  Register1/1 -> ch_out/1
  [mux_sel] -> Gateway Out/1, ST2/1(In)
  [din_ch0_up] -> Gateway Out1/1, ST1/1(In)
  [din_ch1] -> Gateway Out2/1, ST3/1(In)
  [mux_out] -> Gateway Out5/1
  Gateway Out/1 -> D_S3/1
  Gateway Out1/1 -> D_S3/2
  Gateway Out2/1 -> D_S3/3
  Gateway Out5/1 -> D_S3/4
  mux_sel1/1 -> Register1/1, Mux/1, [mux_sel]
  Clock Enable Probe/1 -> mux_sel1/2

== system ddc_bpm_476_066/TDM_monit/ST1 ==
  In : Inport
  Display : Display
  Sample Time : xbsIndex_r4/Sample Time  block_type=sampletime
      settings: infoedit="The Sample Time block reports the normalized sample period of its input.  A signal's normalized sample period is not equivalent to its Simulink absolute sample period.<br><br>Hardware notes: This block is implemented as a constant in hardware."
  X_monit1 : xbsIndex_r4/Gateway Out  inherit_from_input=on  hdl_port=off  timing_constraint=Data Rate  locs_specified=off  LOCs={}  UseAsDAC=off  DACChannel='1'  block_type=gatewayout
      settings: infoedit="Gateway out block.  Converts Xilinx fixed-point or floating-point type inputs into ouputs of type Simulink integer, single, double, or fixed point.<br><br>Hardware notes:  In hardware these blocks become top level output ports or are discarded, depending on how they are configured."
  wires:
  X_monit1/1 -> Display/1
  Sample Time/1 -> X_monit1/1
  In/1 -> Sample Time/1

== system ddc_bpm_476_066/TDM_monit/ST2 ==
  In : Inport
  Display : Display
  Sample Time : xbsIndex_r4/Sample Time  block_type=sampletime
      settings: infoedit="The Sample Time block reports the normalized sample period of its input.  A signal's normalized sample period is not equivalent to its Simulink absolute sample period.<br><br>Hardware notes: This block is implemented as a constant in hardware."
  X_monit1 : xbsIndex_r4/Gateway Out  inherit_from_input=on  hdl_port=off  timing_constraint=Data Rate  locs_specified=off  LOCs={}  UseAsDAC=off  DACChannel='1'  block_type=gatewayout
      settings: infoedit="Gateway out block.  Converts Xilinx fixed-point or floating-point type inputs into ouputs of type Simulink integer, single, double, or fixed point.<br><br>Hardware notes:  In hardware these blocks become top level output ports or are discarded, depending on how they are configured."
  wires:
  X_monit1/1 -> Display/1
  Sample Time/1 -> X_monit1/1
  In/1 -> Sample Time/1

== system ddc_bpm_476_066/TDM_monit/ST3 ==
  In : Inport
  Display : Display
  Sample Time : xbsIndex_r4/Sample Time  block_type=sampletime
      settings: infoedit="The Sample Time block reports the normalized sample period of its input.  A signal's normalized sample period is not equivalent to its Simulink absolute sample period.<br><br>Hardware notes: This block is implemented as a constant in hardware."
  X_monit1 : xbsIndex_r4/Gateway Out  inherit_from_input=on  hdl_port=off  timing_constraint=Data Rate  locs_specified=off  LOCs={}  UseAsDAC=off  DACChannel='1'  block_type=gatewayout
      settings: infoedit="Gateway out block.  Converts Xilinx fixed-point or floating-point type inputs into ouputs of type Simulink integer, single, double, or fixed point.<br><br>Hardware notes:  In hardware these blocks become top level output ports or are discarded, depending on how they are configured."
  wires:
  X_monit1/1 -> Display/1
  Sample Time/1 -> X_monit1/1
  In/1 -> Sample Time/1

== system ddc_bpm_476_066/TDM_monit/ST5 ==
  In : Inport
  Display : Display
  Sample Time : xbsIndex_r4/Sample Time  block_type=sampletime
      settings: infoedit="The Sample Time block reports the normalized sample period of its input.  A signal's normalized sample period is not equivalent to its Simulink absolute sample period.<br><br>Hardware notes: This block is implemented as a constant in hardware."
  out : xbsIndex_r4/Gateway Out  inherit_from_input=on  hdl_port=off  timing_constraint=Data Rate  locs_specified=off  LOCs={}  UseAsDAC=off  DACChannel='1'  block_type=gatewayout
      settings: infoedit="Gateway out block.  Converts Xilinx fixed-point or floating-point type inputs into ouputs of type Simulink integer, single, double, or fixed point.<br><br>Hardware notes:  In hardware these blocks become top level output ports or are discarded, depending on how they are configured."
  wires:
  out/1 -> Display/1
  Sample Time/1 -> out/1
  In/1 -> Sample Time/1

== system ddc_bpm_476_066/TDM_monit/ST7 ==
  In : Inport
  Display : Display
  Sample Time : xbsIndex_r4/Sample Time  block_type=sampletime
      settings: infoedit="The Sample Time block reports the normalized sample period of its input.  A signal's normalized sample period is not equivalent to its Simulink absolute sample period.<br><br>Hardware notes: This block is implemented as a constant in hardware."
  out : xbsIndex_r4/Gateway Out  inherit_from_input=on  hdl_port=off  timing_constraint=Data Rate  locs_specified=off  LOCs={}  UseAsDAC=off  DACChannel='1'  block_type=gatewayout
      settings: infoedit="Gateway out block.  Converts Xilinx fixed-point or floating-point type inputs into ouputs of type Simulink integer, single, double, or fixed point.<br><br>Hardware notes:  In hardware these blocks become top level output ports or are discarded, depending on how they are configured."
  wires:
  out/1 -> Display/1
  Sample Time/1 -> out/1
  In/1 -> Sample Time/1
